simulink model "KitGewerk2_v1_4"  (R2014a)
settings: Solver=ode3  StartTime=0.0  StopTime=inf  FixedStep=0.005  RelTol=1e-3
undefined symbols (not defined in the file or in its folder): Com1, none
libraries: slrtlib x14, dspswit3 x1, xpcseriallib x1
(part 1 of 2)
CloseFcn:
  | rtwprivate ssgencode ModelCloseRequest Robotino_Strecke_reall_2009
settings Model: SimulationMode=external  BufferReuse=off  Creator=atlabor  LastModifiedBy=atlabor
settings SolverCC: EnableConcurrentExecution=on
settings DataIOCC: LimitDataPoints=off  SignalLoggingSaveFormat=ModelDataLogs
settings OptimizationCC: BlockReduction=off  OptimizeBlockIOStorage=off  BufferReuse=off  GlobalBufferReuse=off  ExpressionFolding=off  ExpressionDepthLimit=2147483647  LocalBlockOutputs=off  InitFltsAndDblsToZero=on
settings DebuggingCC: SaveWithParameterizedLinksMsg=none  UnderspecifiedInitializationDetection=Classic  FcnCallInpInsideContextMsg=UseLocalSettings  StateNameClashWarn=warning
settings HardwareCC: ProdIntDivRoundTo=Zero  ProdEndianess=LittleEndian  ProdHWDeviceType=Generic->32-bit x86 compatible
settings SFSimCC: SimParseCustomCode=off
settings RTWCC: SystemTargetFile=slrt.tlc  TemplateMakefile=slrt_default_tmf  Description=Simulink Real-Time  ProcessScript=slrt_make_rtw_hook  RTWCompilerOptimization=On
settings SimulinkRealTimeCC: GeneratePreprocessorConditionals=Disable all  EnableShiftOperators=on

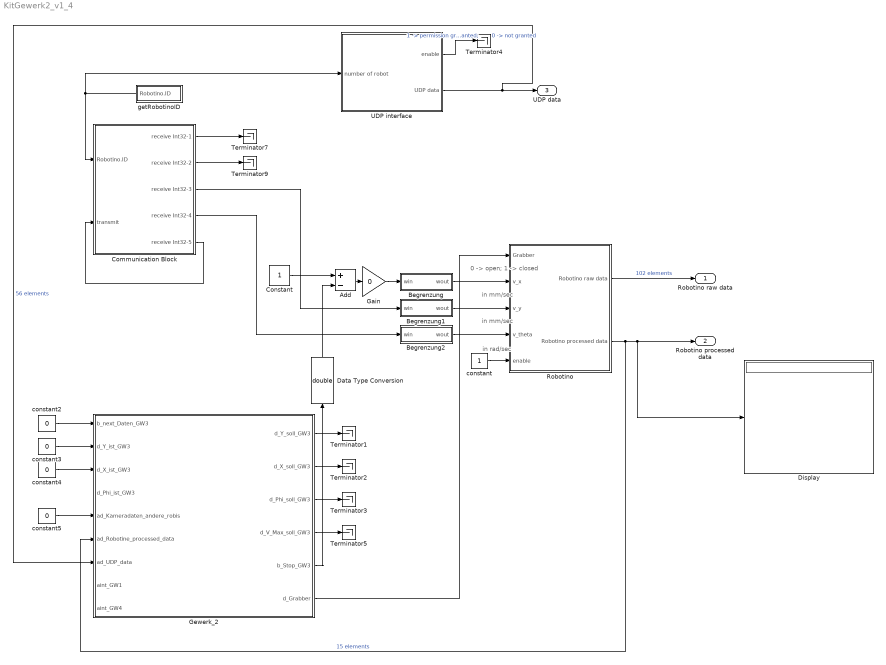
== system KitGewerk2_v1_4 ==
  note: 0 -> open; 1 -> closed
  note: in rad/sec
  note: in mm/sec
  note: in mm/sec
  Add : Sum  Inputs=+-
  Begrenzung : MATLAB Function  TreatAsAtomicUnit=on
  Begrenzung1 : MATLAB Function  TreatAsAtomicUnit=on
  Begrenzung2 : MATLAB Function  TreatAsAtomicUnit=on
  Communication Block : Subsystem
  Constant : Constant
  Data Type Conversion : DataTypeConversion  OutDataTypeStr=double
  Display : Display
  Gain : Gain  Gain=0
  Gewerk_2 : Subsystem
  Robotino : Subsystem
  Terminator{1..5,7,9} (7 alike) : Terminator
  UDP interface : Subsystem
  constant : Constant
  constant2 : Constant  Value=0  OutDataTypeStr=boolean
  constant3 : Constant  Value=0  OutDataTypeStr=double
  constant4 : Constant  Value=0
  constant5 : Constant  Value=0
  getRobotinoID : Subsystem
  Robotino raw data : Outport
  Robotino processed data : Outport  Port=2
  UDP data : Outport  Port=3
  wires:
  Robotino/1(Robotino raw data) -> Robotino raw data/1  "102 elements"
  Begrenzung1/1(wout) -> Robotino/3(v_y)
  Begrenzung/1(wout) -> Robotino/2(v_x)
  Communication Block/2(receive Int32-2) -> Terminator9/1
  UDP interface/1(enable) -> Terminator4/1  "1 -> permission granted;        0 -> not granted"
  constant/1 -> Robotino/5(enable)
  getRobotinoID/1(Robotino.ID) -> UDP interface/1(number of robot), Communication Block/1(Robotino.ID)
  Communication Block/5(receive Int32-5) -> Communication Block/2(transmit)
  Begrenzung2/1(wout) -> Robotino/4(v_theta)
  UDP interface/2(UDP data) -> Gewerk_2/7(ad_UDP_data), UDP data/1  "56 elements"
  Robotino/2(Robotino processed data) -> Gewerk_2/6(ad_Robotine_processed_data), Display/1, Robotino processed data/1  "15 elements"
  constant3/1 -> Gewerk_2/2(d_Y_ist_GW3)
  constant4/1 -> Gewerk_2/3(d_X_ist_GW3)
  constant5/1 -> Gewerk_2/5(ad_Kameradaten_andere_robis)
  Communication Block/3(receive Int32-3) -> Begrenzung1/1(win)
  Communication Block/4(receive Int32-4) -> Begrenzung2/1(win)
  Gewerk_2/1(d_Y_soll_GW3) -> Terminator1/1
  Gewerk_2/2(d_X_soll_GW3) -> Terminator2/1
  Gewerk_2/3(d_Phi_soll_GW3) -> Terminator3/1
  Gewerk_2/4(d_V_Max_soll_GW3) -> Terminator5/1
  Communication Block/1(receive Int32-1) -> Terminator7/1
  Add/1 -> Gain/1
  Constant/1 -> Add/1
  constant2/1 -> Gewerk_2/1(b_next_Daten_GW3)
  Gain/1 -> Begrenzung/1(win)
  Gewerk_2/5(b_Stop_GW3) -> Data Type Conversion/1
  Gewerk_2/6(d_Grabber) -> Robotino/1(Grabber)
  Data Type Conversion/1 -> Add/2

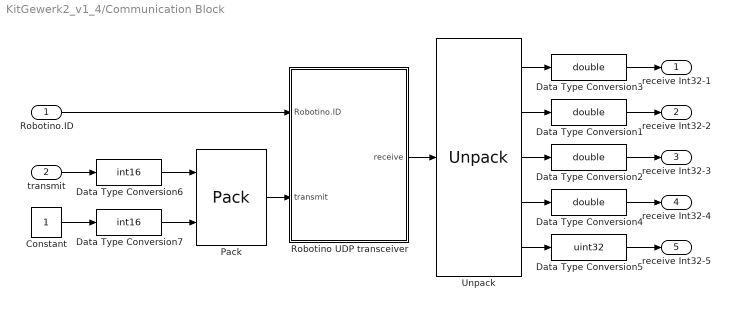
== system KitGewerk2_v1_4/Communication Block ==
  Robotino.ID : Inport
  transmit : Inport  Port=2
  Constant : Constant
  Data Type Conversion{1..4} (4 alike) : DataTypeConversion  OutDataTypeStr=double
  Data Type Conversion5 : DataTypeConversion  OutDataTypeStr=uint32
  Data Type Conversion6 : DataTypeConversion  OutDataTypeStr=int16
  Data Type Conversion7 : DataTypeConversion  OutDataTypeStr=int16
  Pack : slrtlib/UDP/Pack   datatypes={'int16','int16'}  byteAlign=1
  Robotino UDP transceiver : Subsystem
  Unpack : slrtlib/UDP/Unpack   dimensions={1, 1, 1, 1, 1}  datatypes={'int32','int32','int32','int32','int32'}  byteAlign=1
  receive Int32-1 : Outport
  receive Int32-2 : Outport  Port=2
  receive Int32-3 : Outport  Port=3
  receive Int32-4 : Outport  Port=4
  receive Int32-5 : Outport  Port=5
  wires:
  Unpack/1 -> Data Type Conversion3/1
  Unpack/5 -> Data Type Conversion5/1
  Unpack/2 -> Data Type Conversion1/1
  Unpack/3 -> Data Type Conversion2/1
  Unpack/4 -> Data Type Conversion4/1
  Data Type Conversion1/1 -> receive Int32-2/1
  Data Type Conversion2/1 -> receive Int32-3/1
  Data Type Conversion3/1 -> receive Int32-1/1
  Data Type Conversion4/1 -> receive Int32-4/1
  Data Type Conversion5/1 -> receive Int32-5/1
  transmit/1 -> Data Type Conversion6/1
  Pack/1 -> Robotino UDP transceiver/2(transmit)
  Data Type Conversion6/1 -> Pack/1
  Data Type Conversion7/1 -> Pack/2
  Constant/1 -> Data Type Conversion7/1
  Robotino.ID/1 -> Robotino UDP transceiver/1(Robotino.ID)
  Robotino UDP transceiver/1(receive) -> Unpack/1

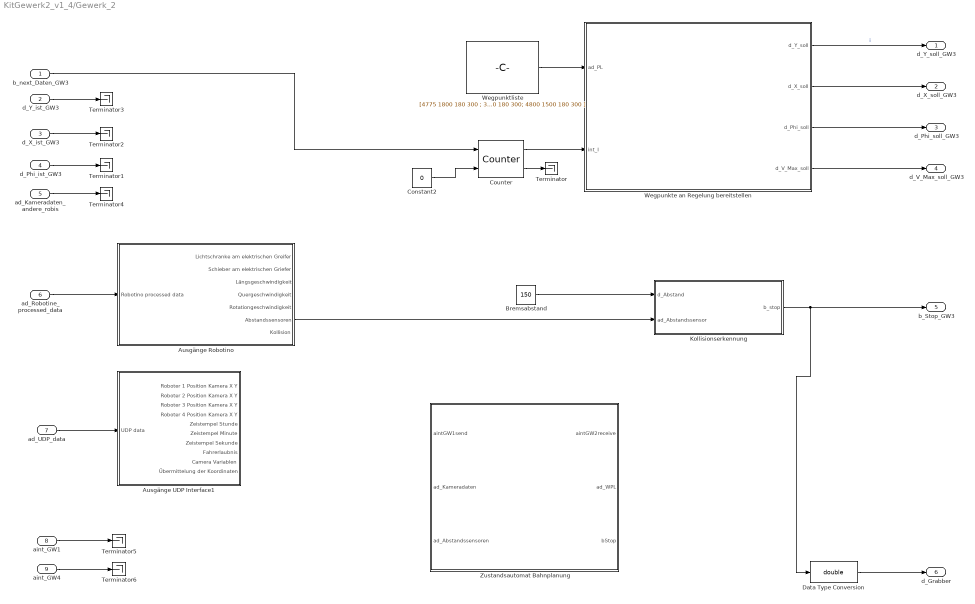
== system KitGewerk2_v1_4/Gewerk_2 ==
  b_next_Daten_GW3 : Inport  OutDataTypeStr=boolean
  d_Y_ist_GW3 : Inport  Port=2  OutDataTypeStr=double
  d_X_ist_GW3 : Inport  Port=3  OutDataTypeStr=double
  d_Phi_ist_GW3 : Inport  Port=4  OutDataTypeStr=double
  ad_Kameradaten_andere_robis : Inport  Port=5  OutDataTypeStr=double
  ad_Robotine_processed_data : Inport  Port=6
  ad_UDP_data : Inport  Port=7  OutDataTypeStr=double
  aint_GW1 : Inport  Port=8  OutDataTypeStr=boolean
  aint_GW4 : Inport  Port=9  OutDataTypeStr=boolean
  Ausgänge Robotino : Subsystem
  Ausgänge UDP Interface1 : Subsystem
  Bremsabstand : Constant  Value=150  OutDataTypeStr=double
  Constant2 : Constant  Value=0
  Counter : dspswit3/Counter  Direction=Up  CountEvent=Rising edge  CounterSize=User defined  MaxCount=16  InitialCount=0  Output=Count and Hit  HitValue=16  ResetInput=on  SamplesPerFrame=1  Ts=1  CntDtype=int32  HitDtype=Logical
  Data Type Conversion : DataTypeConversion  OutDataTypeStr=double
  Kollisionserkennung : MATLAB Function  TreatAsAtomicUnit=on
  Terminator{,1..6} (7 alike) : Terminator
  Wegpunkte an Regelung bereitstellen : MATLAB Function  TreatAsAtomicUnit=on
  Wegpunktliste : Constant  Value=[4775 1800 180 300 ; 3745 1800 180 300; 2540 2100 180 300; 2160 2100 180 300; 1678 1894 180 300; 1373 1846 180 300; 1155 1627 180 300; 1106 1321 180 300; 1246 1046 180 300; 1522 906 180 300; 1827 954 180 300; 2300 954 180 300; 2800 1500 180 300; 3300 1000 180 300; 3800 1500 180 300; 4300 1000 180 300; 4800 1500 180 300 ]  OutDataTypeStr=double
  Zustandsautomat Bahnplanung : Stateflow chart  TreatAsAtomicUnit=on
  d_Y_soll_GW3 : Outport  OutDataTypeStr=double
  d_X_soll_GW3 : Outport  Port=2  OutDataTypeStr=double
  d_Phi_soll_GW3 : Outport  Port=3  OutDataTypeStr=double
  d_V_Max_soll_GW3 : Outport  Port=4  OutDataTypeStr=double
  b_Stop_GW3 : Outport  Port=5  OutDataTypeStr=boolean
  d_Grabber : Outport  Port=6  OutDataTypeStr=double
  wires:
  d_Y_ist_GW3/1 -> Terminator3/1
  ad_Kameradaten_andere_robis/1 -> Terminator4/1
  d_Phi_ist_GW3/1 -> Terminator1/1
  d_X_ist_GW3/1 -> Terminator2/1
  Wegpunktliste/1 -> Wegpunkte an Regelung bereitstellen/1(ad_PL)
  Counter/1 -> Wegpunkte an Regelung bereitstellen/2(int_I)
  Wegpunkte an Regelung bereitstellen/2(d_X_soll) -> d_X_soll_GW3/1
  b_next_Daten_GW3/1 -> Counter/1
  Wegpunkte an Regelung bereitstellen/1(d_Y_soll) -> d_Y_soll_GW3/1  "i"
  Wegpunkte an Regelung bereitstellen/4(d_V_Max_soll) -> d_V_Max_soll_GW3/1
  Wegpunkte an Regelung bereitstellen/3(d_Phi_soll) -> d_Phi_soll_GW3/1
  Constant2/1 -> Counter/2
  Counter/2 -> Terminator/1
  Kollisionserkennung/1(b_stop) -> Data Type Conversion/1, b_Stop_GW3/1
  Ausgänge Robotino/6(Abstandssensoren) -> Kollisionserkennung/2(ad_Abstandssensor)
  Bremsabstand/1 -> Kollisionserkennung/1(d_Abstand)
  ad_Robotine_processed_data/1 -> Ausgänge Robotino/1(Robotino processed data)
  ad_UDP_data/1 -> Ausgänge UDP Interface1/1(UDP data)
  Data Type Conversion/1 -> d_Grabber/1
  aint_GW4/1 -> Terminator6/1
  aint_GW1/1 -> Terminator5/1

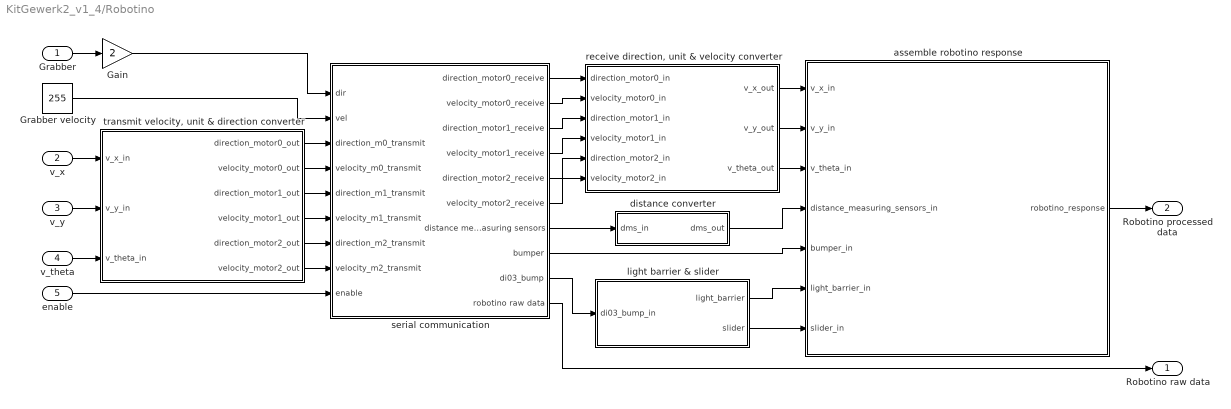
== system KitGewerk2_v1_4/Robotino ==
  Grabber : Inport
  v_x : Inport  Port=2
  v_y : Inport  Port=3
  v_theta : Inport  Port=4
  enable : Inport  Port=5
  Gain : Gain  Gain=2
  Grabber velocity : Constant  Value=255
  assemble robotino response : MATLAB Function  TreatAsAtomicUnit=on
  distance converter : MATLAB Function  TreatAsAtomicUnit=on
  light barrier & slider : MATLAB Function  TreatAsAtomicUnit=on
  "receive direction, unit & velocity converter" : MATLAB Function  TreatAsAtomicUnit=on
  serial communication : Subsystem
  "transmit velocity, unit & direction converter" : MATLAB Function  TreatAsAtomicUnit=on
  Robotino raw data : Outport
  Robotino processed data : Outport  Port=2
  wires:
  "transmit velocity, unit & direction converter"/1(direction_motor0_out) -> serial communication/3(direction_m0_transmit)
  "transmit velocity, unit & direction converter"/2(velocity_motor0_out) -> serial communication/4(velocity_m0_transmit)
  "transmit velocity, unit & direction converter"/3(direction_motor1_out) -> serial communication/5(direction_m1_transmit)
  "transmit velocity, unit & direction converter"/4(velocity_motor1_out) -> serial communication/6(velocity_m1_transmit)
  "transmit velocity, unit & direction converter"/5(direction_motor2_out) -> serial communication/7(direction_m2_transmit)
  "transmit velocity, unit & direction converter"/6(velocity_motor2_out) -> serial communication/8(velocity_m2_transmit)
  v_x/1 -> "transmit velocity, unit & direction converter"/1(v_x_in)
  v_y/1 -> "transmit velocity, unit & direction converter"/2(v_y_in)
  v_theta/1 -> "transmit velocity, unit & direction converter"/3(v_theta_in)
  "receive direction, unit & velocity converter"/2(v_y_out) -> assemble robotino response/2(v_y_in)
  enable/1 -> serial communication/9(enable)
  serial communication/1(direction_motor0_receive) -> "receive direction, unit & velocity converter"/1(direction_motor0_in)
  serial communication/7(distance measuring sensors) -> distance converter/1(dms_in)
  serial communication/10(robotino raw data) -> Robotino raw data/1
  serial communication/9(di03_bump) -> light barrier & slider/1(di03_bump_in)
  "receive direction, unit & velocity converter"/1(v_x_out) -> assemble robotino response/1(v_x_in)
  "receive direction, unit & velocity converter"/3(v_theta_out) -> assemble robotino response/3(v_theta_in)
  assemble robotino response/1(robotino_response) -> Robotino processed data/1
  Grabber/1 -> Gain/1
  Gain/1 -> serial communication/1(dir)
  distance converter/1(dms_out) -> assemble robotino response/4(distance_measuring_sensors_in)
  light barrier & slider/2(slider) -> assemble robotino response/7(slider_in)
  light barrier & slider/1(light_barrier) -> assemble robotino response/6(light_barrier_in)
  serial communication/8(bumper) -> assemble robotino response/5(bumper_in)
  serial communication/2(velocity_motor0_receive) -> "receive direction, unit & velocity converter"/2(velocity_motor0_in)
  serial communication/3(direction_motor1_receive) -> "receive direction, unit & velocity converter"/3(direction_motor1_in)
  serial communication/4(velocity_motor1_receive) -> "receive direction, unit & velocity converter"/4(velocity_motor1_in)
  serial communication/5(direction_motor2_receive) -> "receive direction, unit & velocity converter"/5(direction_motor2_in)
  serial communication/6(velocity_motor2_receive) -> "receive direction, unit & velocity converter"/6(velocity_motor2_in)
  Grabber velocity/1 -> serial communication/2(vel)

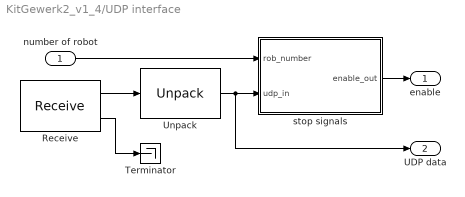
== system KitGewerk2_v1_4/UDP interface ==
  number of robot : Inport
  Receive : slrtlib/UDP/Receive   ipAddress=0.0.0.0  ipPort=25000  width=448  vblLen=off  sampletime=-1
  Terminator : Terminator
  Unpack : slrtlib/UDP/Unpack   dimensions={[56]}  datatypes={'double'}  byteAlign=1
  stop signals : MATLAB Function  TreatAsAtomicUnit=on
  enable : Outport
  UDP data : Outport  Port=2
  wires:
  Unpack/1 -> stop signals/2(udp_in), UDP data/1
  Receive/1 -> Unpack/1
  Receive/2 -> Terminator/1
  stop signals/1(enable_out) -> enable/1
  number of robot/1 -> stop signals/1(rob_number)

== system KitGewerk2_v1_4/getRobotinoID ==
  note: Executing only once at start after 10ms
  Step : Step  Time=0.01  SampleTime=0
  getIDfromFlash : Subsystem
  Robotino.ID : Outport
  wires:
  Step/1 -> getIDfromFlash/Trigger
  getIDfromFlash/1(RobotinoID) -> Robotino.ID/1

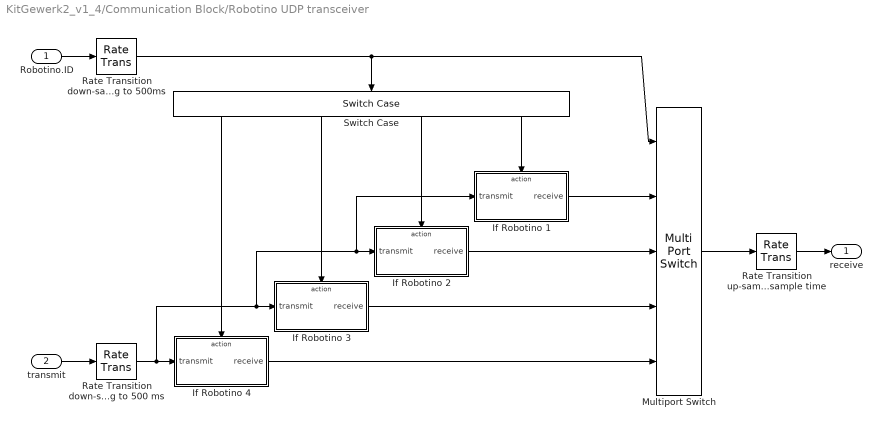
== system KitGewerk2_v1_4/Communication Block/Robotino UDP transceiver ==
  Robotino.ID : Inport
  transmit : Inport  Port=2
  If Robotino 1 : Subsystem  TreatAsAtomicUnit=on
  If Robotino 2 : Subsystem  TreatAsAtomicUnit=on
  If Robotino 3 : Subsystem  TreatAsAtomicUnit=on
  If Robotino 4 : Subsystem  TreatAsAtomicUnit=on
  Multiport Switch : MultiPortSwitch  Inputs=4
  Rate Transition down-sampling to 500 ms : RateTransition  OutPortSampleTime=0.5
  Rate Transition down-sampling to 500ms : RateTransition  OutPortSampleTime=0.5
  Rate Transition up-sampling to fundamental sample time : RateTransition
  Switch Case : SwitchCase  CaseConditions={4,3,2,1}  ShowDefaultCase=off
  receive : Outport
  wires:
  Switch Case/1 -> If Robotino 4/Action
  Switch Case/2 -> If Robotino 3/Action
  Switch Case/3 -> If Robotino 2/Action
  Switch Case/4 -> If Robotino 1/Action
  Multiport Switch/1 -> Rate Transition up-sampling to fundamental sample time/1
  If Robotino 1/1(receive) -> Multiport Switch/2
  If Robotino 3/1(receive) -> Multiport Switch/4
  If Robotino 2/1(receive) -> Multiport Switch/3
  If Robotino 4/1(receive) -> Multiport Switch/5
  transmit/1 -> Rate Transition down-sampling to 500 ms/1
  Rate Transition up-sampling to fundamental sample time/1 -> receive/1
  Rate Transition down-sampling to 500 ms/1 -> If Robotino 4/1(transmit), If Robotino 3/1(transmit), If Robotino 2/1(transmit), If Robotino 1/1(transmit)
  Robotino.ID/1 -> Rate Transition down-sampling to 500ms/1
  Rate Transition down-sampling to 500ms/1 -> Switch Case/1, Multiport Switch/1

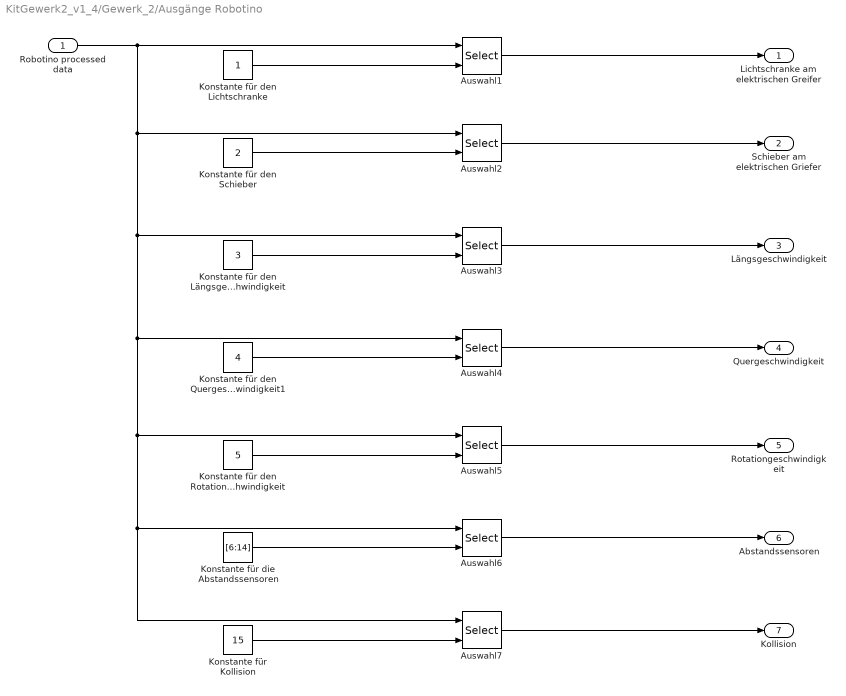
== system KitGewerk2_v1_4/Gewerk_2/Ausgänge Robotino ==
  Robotino processed data : Inport
  Auswahl{1..7} (7 alike) : Selector  InputPortWidth=15  IndexOptions=Index vector (port)  Indices=[1 3]
  "Konstante für Kollision " : Constant  Value=15
  Konstante für den Lichtschranke : Constant
  Konstante für den Längsgeschwindigkeit : Constant  Value=3
  Konstante für den Quergeschwindigkeit1 : Constant  Value=4
  Konstante für den Rotationegeschwindigkeit : Constant  Value=5
  Konstante für den Schieber : Constant  Value=2
  Konstante für die Abstandssensoren : Constant  Value=[6:14]
  Lichtschranke am elektrischen Greifer : Outport
  "Schieber am elektrischen Griefer " : Outport  Port=2
  "Längsgeschwindigkeit " : Outport  Port=3
  Quergeschwindigkeit : Outport  Port=4
  "Rotationgeschwindigkeit " : Outport  Port=5
  Abstandssensoren : Outport  Port=6
  Kollision : Outport  Port=7
  wires:
  Auswahl1/1 -> Lichtschranke am elektrischen Greifer/1
  Robotino processed data/1 -> Auswahl1/1, Auswahl5/1, Auswahl7/1, Auswahl6/1, Auswahl4/1, Auswahl3/1, Auswahl2/1
  Konstante für den Lichtschranke/1 -> Auswahl1/2
  Konstante für den Schieber/1 -> Auswahl2/2
  Auswahl2/1 -> "Schieber am elektrischen Griefer "/1
  Konstante für den Längsgeschwindigkeit/1 -> Auswahl3/2
  Auswahl3/1 -> "Längsgeschwindigkeit "/1
  Konstante für den Quergeschwindigkeit1/1 -> Auswahl4/2
  Auswahl4/1 -> Quergeschwindigkeit/1
  Auswahl5/1 -> "Rotationgeschwindigkeit "/1
  Konstante für den Rotationegeschwindigkeit/1 -> Auswahl5/2
  Konstante für die Abstandssensoren/1 -> Auswahl6/2
  Auswahl6/1 -> Abstandssensoren/1
  Auswahl7/1 -> Kollision/1
  "Konstante für Kollision "/1 -> Auswahl7/2

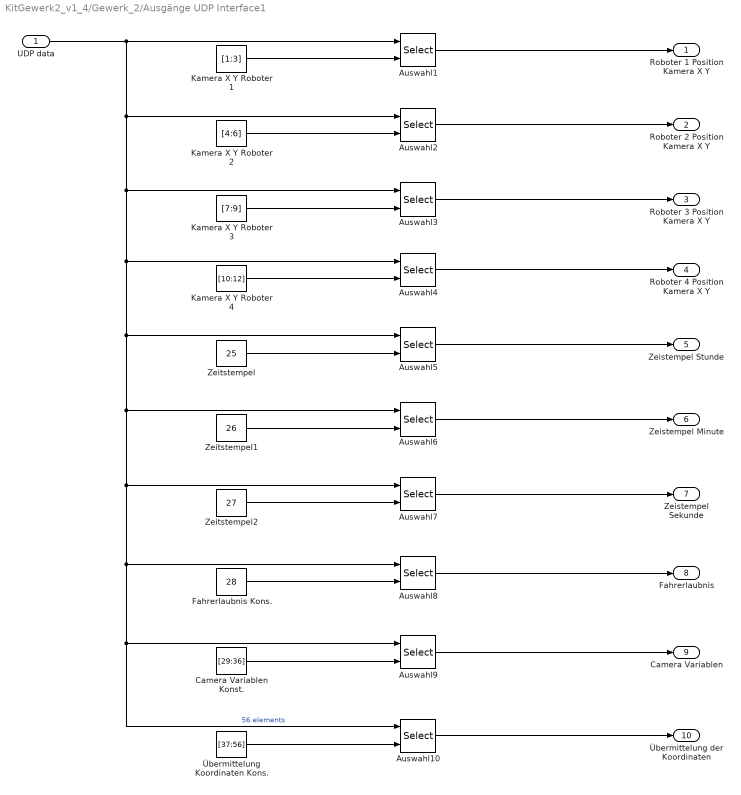
== system KitGewerk2_v1_4/Gewerk_2/Ausgänge UDP Interface1 ==
  UDP data : Inport
  Auswahl{1..10} (10 alike) : Selector  InputPortWidth=56  IndexOptions=Index vector (port)  Indices=[1 3]
  Camera Variablen Konst. : Constant  Value=[29:36]
  Fahrerlaubnis Kons. : Constant  Value=28
  Kamera X Y Roboter 1 : Constant  Value=[1:3]
  Kamera X Y Roboter 2 : Constant  Value=[4:6]
  Kamera X Y Roboter 3 : Constant  Value=[7:9]
  Kamera X Y Roboter 4 : Constant  Value=[10:12]
  Zeitstempel : Constant  Value=25
  Zeitstempel1 : Constant  Value=26
  Zeitstempel2 : Constant  Value=27
  Übermittelung Koordinaten Kons. : Constant  Value=[37:56]
  Roboter 1 Position Kamera X Y : Outport
  Roboter 2 Position Kamera X Y : Outport  Port=2
  Roboter 3 Position Kamera X Y : Outport  Port=3
  Roboter 4 Position Kamera X Y : Outport  Port=4
  Zeistempel Stunde : Outport  Port=5
  Zeistempel Minute : Outport  Port=6
  Zeistempel Sekunde : Outport  Port=7
  Fahrerlaubnis : Outport  Port=8
  Camera Variablen : Outport  Port=9
  Übermittelung der Koordinaten : Outport  Port=10
  wires:
  Kamera X Y Roboter 1/1 -> Auswahl1/2
  Kamera X Y Roboter 2/1 -> Auswahl2/2
  Kamera X Y Roboter 3/1 -> Auswahl3/2
  Kamera X Y Roboter 4/1 -> Auswahl4/2
  Auswahl1/1 -> Roboter 1 Position Kamera X Y/1
  Auswahl3/1 -> Roboter 3 Position Kamera X Y/1
  Auswahl2/1 -> Roboter 2 Position Kamera X Y/1
  Auswahl4/1 -> Roboter 4 Position Kamera X Y/1
  Zeitstempel/1 -> Auswahl5/2
  Auswahl5/1 -> Zeistempel Stunde/1
  Zeitstempel1/1 -> Auswahl6/2
  Auswahl6/1 -> Zeistempel Minute/1
  Zeitstempel2/1 -> Auswahl7/2
  Auswahl7/1 -> Zeistempel Sekunde/1
  Fahrerlaubnis Kons./1 -> Auswahl8/2
  Auswahl8/1 -> Fahrerlaubnis/1
  Camera Variablen Konst./1 -> Auswahl9/2
  Auswahl9/1 -> Camera Variablen/1
  UDP data/1 -> Auswahl2/1, Auswahl10/1, Auswahl9/1, Auswahl8/1, Auswahl7/1, Auswahl6/1, Auswahl5/1, Auswahl4/1, Auswahl3/1, Auswahl1/1  "56 elements"
  Übermittelung Koordinaten Kons./1 -> Auswahl10/2
  Auswahl10/1 -> Übermittelung der Koordinaten/1

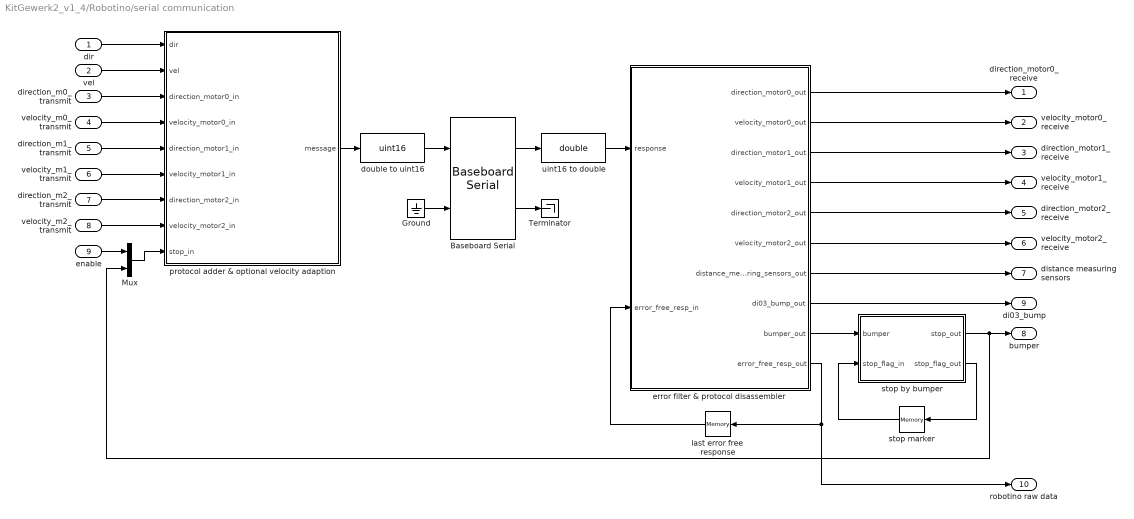
== system KitGewerk2_v1_4/Robotino/serial communication ==
  dir : Inport
  vel : Inport  Port=2
  direction_m0_transmit : Inport  Port=3
  velocity_m0_transmit : Inport  Port=4
  direction_m1_transmit : Inport  Port=5
  velocity_m1_transmit : Inport  Port=6
  direction_m2_transmit : Inport  Port=7
  velocity_m2_transmit : Inport  Port=8
  enable : Inport  Port=9
  Baseboard Serial : xpcseriallib/Mainboard/Baseboard Serial  group=Transmit Setup  port=2  irqnum=4  saddr1=0x3f8  saddr2=0x3e8  config=Com1/none  baud1=115200  parity1=None  ndata1=8  nstop1=1  fifomode1=16 deep  rlevel1=almost full  automode1=off  xmtfifosize1=10240  xmtdatatype1=count+16 bit uint  rcvfifosize1=10240  rcvmaxread1=101  rcvminread1=1  rcvusedelim1=on  rcvdelim1=99  rcvdatatype1=count+16 bit uint  rcvsampletime1=-1  baud2=115200  parity2=None  ndata2=8  nstop2=1  fifomode2=16 deep  rlevel2=almost full  automode2=off  xmtfifosize2=10240  xmtdatatype2=count+16 bit uint  rcvfifosize2=10240  rcvmaxread2=101  rcvminread2=1  rcvusedelim2=on  rcvdelim2=99  rcvdatatype2=count+16 bit uint  rcvsampletime2=-1
      link override FIFO read 1: maxsize=101  minsize=1  usedelimiter=on  delimiter=99  outputtype=count+16 bit uint  sampletime=dt / 2
      link override FIFO read 2: maxsize=101  minsize=1  usedelimiter=on  delimiter=99  outputtype=count+16 bit uint  sampletime=dt / 2
      link override FIFO write 1: size=1024  inputtype=count+16 bit uint  sampletime=-1  id=XMT channel 1, IRQ 4
      link override FIFO write 2: size=1024  inputtype=8 bit uint null terminated  id=XMT channel 2, IRQ 4
      link override Setup1: baud=115200  width=8  nstop=1  parity=None  fmode=16 deep  rlevel=half full  ctsmode=off
      link override Setup2: baud=4800  width=8  nstop=1  parity=None  fmode=16 deep  rlevel=half full  ctsmode=off
  Ground : Ground
  Mux : Mux  Inputs=2
  Terminator : Terminator
  double to uint16 : DataTypeConversion  OutDataTypeStr=uint16  RndMeth=Nearest
  error filter & protocol disassembler : MATLAB Function  TreatAsAtomicUnit=on
  last error free response : Memory  X0=[zeros(1,102)]
  protocol adder & optional velocity adaption : MATLAB Function  TreatAsAtomicUnit=on
  stop by bumper : MATLAB Function  TreatAsAtomicUnit=on
  stop marker : Memory  X0=[zeros(1,3)]
  uint16 to double : DataTypeConversion  OutDataTypeStr=double  RndMeth=Nearest
  direction_motor0_receive : Outport
  velocity_motor0_receive : Outport  Port=2
  direction_motor1_receive : Outport  Port=3
  velocity_motor1_receive : Outport  Port=4
  direction_motor2_receive : Outport  Port=5
  velocity_motor2_receive : Outport  Port=6
  distance measuring sensors : Outport  Port=7
  bumper : Outport  Port=8
  di03_bump : Outport  Port=9
  robotino raw data : Outport  Port=10
  wires:
  Ground/1 -> Baseboard Serial/2
  Baseboard Serial/2 -> Terminator/1
  double to uint16/1 -> Baseboard Serial/1
  protocol adder & optional velocity adaption/1(message) -> double to uint16/1
  stop marker/1 -> stop by bumper/2(stop_flag_in)
  stop by bumper/2(stop_flag_out) -> stop marker/1
  last error free response/1 -> error filter & protocol disassembler/2(error_free_resp_in)
  error filter & protocol disassembler/10(error_free_resp_out) -> last error free response/1, robotino raw data/1
  error filter & protocol disassembler/1(direction_motor0_out) -> direction_motor0_receive/1
  error filter & protocol disassembler/2(velocity_motor0_out) -> velocity_motor0_receive/1
  error filter & protocol disassembler/3(direction_motor1_out) -> direction_motor1_receive/1
  error filter & protocol disassembler/4(velocity_motor1_out) -> velocity_motor1_receive/1
  direction_m0_transmit/1 -> protocol adder & optional velocity adaption/3(direction_motor0_in)
  error filter & protocol disassembler/5(direction_motor2_out) -> direction_motor2_receive/1
  velocity_m0_transmit/1 -> protocol adder & optional velocity adaption/4(velocity_motor0_in)
  error filter & protocol disassembler/6(velocity_motor2_out) -> velocity_motor2_receive/1
  direction_m1_transmit/1 -> protocol adder & optional velocity adaption/5(direction_motor1_in)
  velocity_m1_transmit/1 -> protocol adder & optional velocity adaption/6(velocity_motor1_in)
  direction_m2_transmit/1 -> protocol adder & optional velocity adaption/7(direction_motor2_in)
  velocity_m2_transmit/1 -> protocol adder & optional velocity adaption/8(velocity_motor2_in)
  error filter & protocol disassembler/9(bumper_out) -> stop by bumper/1(bumper)
  stop by bumper/1(stop_out) -> bumper/1, Mux/2
  error filter & protocol disassembler/7(distance_measuring_sensors_out) -> distance measuring sensors/1
  Baseboard Serial/1 -> uint16 to double/1
  uint16 to double/1 -> error filter & protocol disassembler/1(response)
  enable/1 -> Mux/1
  dir/1 -> protocol adder & optional velocity adaption/1(dir)
  vel/1 -> protocol adder & optional velocity adaption/2(vel)
  Mux/1 -> protocol adder & optional velocity adaption/9(stop_in)
  error filter & protocol disassembler/8(di03_bump_out) -> di03_bump/1

== system KitGewerk2_v1_4/getRobotinoID/getIDfromFlash ==
  Trigger : TriggerPort
  From File : slrtlib/Target Management/From File   filename='robotino.id'  dataSize=8  bufSize=2000  readSize=512  EOFOption=Seek to beginning  sampTime=-1  show2ports=off
  Unpack : slrtlib/UDP/Unpack   dimensions={[1]}  datatypes={'double'}  byteAlign=1
  RobotinoID : Outport
  wires:
  From File/1 -> Unpack/1
  Unpack/1 -> RobotinoID/1

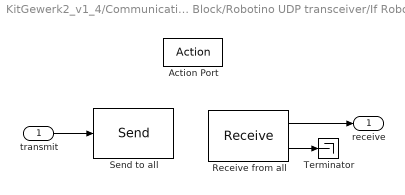
== system KitGewerk2_v1_4/Communication Block/Robotino UDP transceiver/If Robotino 1 ==
  transmit : Inport
  Action Port : ActionPort  ActionType=case
  Receive from all : slrtlib/UDP/Receive   ipAddress=0.0.0.0  ipPort=25011  width=20  vblLen=off  sampletime=-1
  Send to all : slrtlib/UDP/Send   ipAddress=255.255.255.255  ipPort=25010  localPort=-1  vblLen=off  sampletime=-1
  Terminator : Terminator
  receive : Outport
  wires:
  Receive from all/1 -> receive/1
  Receive from all/2 -> Terminator/1
  transmit/1 -> Send to all/1

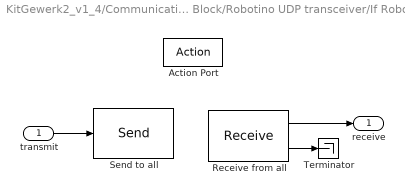
== system KitGewerk2_v1_4/Communication Block/Robotino UDP transceiver/If Robotino 2 ==
  transmit : Inport
  Action Port : ActionPort  ActionType=case
  Receive from all : slrtlib/UDP/Receive   ipAddress=0.0.0.0  ipPort=25012  width=20  vblLen=off  sampletime=-1
  Send to all : slrtlib/UDP/Send   ipAddress=255.255.255.255  ipPort=25020  localPort=-1  vblLen=off  sampletime=-1
  Terminator : Terminator
  receive : Outport
  wires:
  Receive from all/1 -> receive/1
  Receive from all/2 -> Terminator/1
  transmit/1 -> Send to all/1

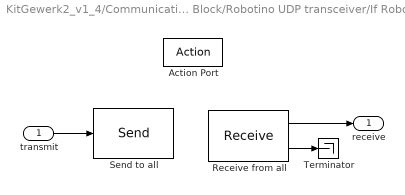
== system KitGewerk2_v1_4/Communication Block/Robotino UDP transceiver/If Robotino 3 ==
  transmit : Inport
  Action Port : ActionPort  ActionType=case
  Receive from all : slrtlib/UDP/Receive   ipAddress=0.0.0.0  ipPort=25013  width=20  vblLen=off  sampletime=-1
  Send to all : slrtlib/UDP/Send   ipAddress=255.255.255.255  ipPort=25030  localPort=-1  vblLen=off  sampletime=-1
  Terminator : Terminator
  receive : Outport
  wires:
  Receive from all/1 -> receive/1
  Receive from all/2 -> Terminator/1
  transmit/1 -> Send to all/1

== system KitGewerk2_v1_4/Communication Block/Robotino UDP transceiver/If Robotino 4 ==
  transmit : Inport
  Action Port : ActionPort  ActionType=case
  Receive from all : slrtlib/UDP/Receive   ipAddress=0.0.0.0  ipPort=25014  width=20  vblLen=off  sampletime=-1
  Send to all : slrtlib/UDP/Send   ipAddress=255.255.255.255  ipPort=25040  localPort=-1  vblLen=off  sampletime=-1
  Terminator : Terminator
  receive : Outport
  wires:
  Receive from all/1 -> receive/1
  Receive from all/2 -> Terminator/1
  transmit/1 -> Send to all/1

== matlab function KitGewerk2_v1_4/Robotino/transmit velocity, unit & direction converter ==
  settings: sampleTime=2*dtpc
  data: direction_motor0_out output; velocity_motor0_out output; direction_motor1_out output; velocity_motor1_out output; direction_motor2_out output; velocity_motor2_out output; v_x_in input; v_y_in input; v_theta_in input
%%%%%%%%%%%%%%%%%%%%%%%%%%%%%%%%%%%%%%%%%%%%%%%%%%%%%%%%%%%%%%%%%%%%%%%%%%%
% conversion from positive and/or negative longitudinal, lateral and      %
% rotational velocities (in milimeters per second) to three separate      %
% positive motor velocities (resolution: 1Byte) and their rotation        %
% direction                                                               %
%                                                                         %
% inputs:  v_x_in (longitudinal velocity in milimeters per second),       %
%          v_y_in (lateral velocity in milimeters per second),            %
%          v_theta_in (rotational velocity in milimeters per second)      %
% outputs: direction_motor0_out (rotating direction of motor0             %
%          (0 := counter-clockwise; 2 := clockwise)),                     %
%          velocity_motor0_out (from 0 to 255),                           %
%          direction_motor1_out (rotating direction of motor1             %
%          (0 := counter-clockwise; 2 := clockwise)),                     %
%          velocity_motor1_out (from 0 to 255),                           %
%          direction_motor2_out (rotating direction of motor2             %
%          (0 := counter-clockwise; 2 := clockwise)),                     %
%          velocity_motor2_out (from 0 to 255)                            %
%%%%%%%%%%%%%%%%%%%%%%%%%%%%%%%%%%%%%%%%%%%%%%%%%%%%%%%%%%%%%%%%%%%%%%%%%%%
function [direction_motor0_out, velocity_motor0_out, ...
          direction_motor1_out, velocity_motor1_out, ...
          direction_motor2_out, velocity_motor2_out] ...
                                          = fcn(v_x_in, v_y_in, v_theta_in)
%%%%%%%%%%%%%%%%%%%%%%%%%%%%%%%%%%%%%%%%%%%%%%%%%%%%%%%%%%%%%%%%%%%%%%
% conversion from longitudinal, lateral & rotational velocity to the %
% three separate motor velocities                                    %
%%%%%%%%%%%%%%%%%%%%%%%%%%%%%%%%%%%%%%%%%%%%%%%%%%%%%%%%%%%%%%%%%%%%%%
v0 = (-v_x_in * cosd(30)) + ( v_y_in * cosd(60)) + (v_theta_in * 135);
v1 =                      + (-v_y_in)            + (v_theta_in * 135);
v2 = ( v_x_in * cosd(30)) + ( v_y_in * cosd(60)) + (v_theta_in * 135);

%%%%%%%%%%%%%%%%%%%%%%%%%%%%%%%%%%%%%%%%%%%%%%%%%%%%%%%%%%%%%%%%%%%%%
% conversion of the separate motor velocities from millimeters to a %
% value between -255 and 255                                        %
%%%%%%%%%%%%%%%%%%%%%%%%%%%%%%%%%%%%%%%%%%%%%%%%%%%%%%%%%%%%%%%%%%%%%
f = 1 / 7.02;
v0 = v0 * f;
v1 = v1 * f;
v2 = v2 * f;

%%%%%%%%%%%%%%%%%%%%%%%%%%%%%%%%%%%%%%%%%%%%%%%%%%%%%%%%%%%%%%%%%%%%
% division of motor velocities into absolute velocity and rotating %
% direction                                                        %
%%%%%%%%%%%%%%%%%%%%%%%%%%%%%%%%%%%%%%%%%%%%%%%%%%%%%%%%%%%%%%%%%%%%
if v0 < 0
    direction_motor0_out =  0;
    velocity_motor0_out  = -v0;
else
    direction_motor0_out = 2;
    velocity_motor0_out  = v0;
end

if v1 < 0
    direction_motor1_out =  0;
    velocity_motor1_out  = -v1;
else
    direction_motor1_out = 2;
    velocity_motor1_out  = v1;
end

if v2 < 0
    direction_motor2_out =  0;
    velocity_motor2_out  = -v2;
else
    direction_motor2_out = 2;
    velocity_motor2_out  = v2;
end

== matlab function KitGewerk2_v1_4/Robotino/serial communication/protocol adder & optional velocity adaption ==
  settings: sampleTime=2*dtpc
  data: dir input; vel input; direction_motor0_in input; velocity_motor0_in input; direction_motor1_in input; velocity_motor1_in input; direction_motor2_in input; velocity_motor2_in input; stop_in input; message output
%%%%%%%%%%%%%%%%%%%%%%%%%%%%%%%%%%%%%%%%%%%%%%%%%%%%%%%%%%%%%%%%%%%%%%%%%%%
% parameterising the 'PC104 to I/O-Board message' for serial line         %
% communication with control commands for the robotino motors             %
%                                                                         %
% optional: velocity adaption as soon as at least one motor is near the   %
%           speed limit                                                   %
%                                                                         %
% inputs: rotating directions and velocities of the three motors          %
% output: vector containing the 'PC104 to I/O-Board message' for serial   %
%         line communication                                              %
%%%%%%%%%%%%%%%%%%%%%%%%%%%%%%%%%%%%%%%%%%%%%%%%%%%%%%%%%%%%%%%%%%%%%%%%%%%
function message = fcn(dir, vel, direction_motor0_in, velocity_motor0_in, ...
                       direction_motor1_in, velocity_motor1_in, ...
                       direction_motor2_in, velocity_motor2_in, stop_in)
%%%%%%%%%%%%%%%%%%%%%%%%%%%%%%
% optional velocity adaption %
%%%%%%%%%%%%%%%%%%%%%%%%%%%%%%
vmax = 175;                                               % v_motor_dez_max

if velocity_motor0_in > vmax
    velocity_motor0_tf = velocity_motor0_in;
    
    velocity_motor0_in = vmax;
    velocity_motor1_in = vmax * velocity_motor1_in / velocity_motor0_tf;
    velocity_motor2_in = vmax * velocity_motor2_in / velocity_motor0_tf;
end

if velocity_motor1_in > vmax
    velocity_motor1_tf = velocity_motor1_in;
    
    velocity_motor0_in = vmax * velocity_motor0_in / velocity_motor1_tf;
    velocity_motor1_in = vmax;
    velocity_motor2_in = vmax * velocity_motor2_in / velocity_motor1_tf;
end

if velocity_motor2_in > vmax
    velocity_motor2_tf = velocity_motor2_in;
    
    velocity_motor0_in = vmax * velocity_motor0_in / velocity_motor2_tf;
    velocity_motor1_in = vmax * velocity_motor1_in / velocity_motor2_tf;
    velocity_motor2_in = vmax;
end
%%%%%%%%%%%%%%%%%%%%%%%%%%%%%%%%%%%%%%%%%%%%%%%%%%%%%%%%%%%%%%%%%%%%%%
% vector containing the 'PC104 to I/O-Board message' for serial line %
% communication                                                      %
%%%%%%%%%%%%%%%%%%%%%%%%%%%%%%%%%%%%%%%%%%%%%%%%%%%%%%%%%%%%%%%%%%%%%%
message = [47, abs('REC'), 5, min(stop_in), direction_motor0_in, ...
           velocity_motor0_in, zeros(1, 4), 255, 255, 255, ...
           min(stop_in), direction_motor1_in, velocity_motor1_in, ...
           zeros(1, 4), 255, 255, 255, min(stop_in), ...
           direction_motor2_in, velocity_motor2_in, zeros(1, 4), 255, ...
           255, 255, 1, dir, vel, zeros(1, 4), 255, 255, 255, abs('rec')].';

== matlab function KitGewerk2_v1_4/UDP interface/stop signals ==
  data: rob_number input; udp_in input; enable_out output
%%%%%%%%%%%%%%%%%%%%%%%%%%%%%%%%%%%%%%%%%%%%%%%%%%%%%%%%%%%%%%%%%%%%%%%%%%%
% Leads the enable command through. The enable command turns the Robotino %
% inputs to selectable form.                                              %
%                                                                         %
% input: udp_in (vector of 56 elements containing the data sent by the    %
%                camera-model)                                            %
% outputs: enable_out (1 = inputs are in selectable form;                 %
%                      0 = inputs are set to 0)                           %
%          udp_out (vector of 56 elements containing the data sent by the %
%                   camera-model)                                         %
%%%%%%%%%%%%%%%%%%%%%%%%%%%%%%%%%%%%%%%%%%%%%%%%%%%%%%%%%%%%%%%%%%%%%%%%%%%
function enable_out  = fcn(rob_number, udp_in)
enable_out = [0, 0];
if (udp_in(rob_number * 3 - 2) <= 0) && ...
   (udp_in(rob_number * 3 - 1) <= 0) && (udp_in(rob_number * 3) <= 0)
    enable_out(1) = 0;
else
    enable_out(1) = 1;
end
enable_out(2) = udp_in(28);

== matlab function KitGewerk2_v1_4/Robotino/serial communication/error filter & protocol disassembler ==
  settings: sampleTime=dtpc/2
  data: response input; error_free_resp_in input; direction_motor0_out output; velocity_motor0_out output; direction_motor1_out output; velocity_motor1_out output; direction_motor2_out output; velocity_motor2_out output; distance_measuring_sensors_out output; di03_bump_out output; bumper_out output; error_free_resp_out output
%%%%%%%%%%%%%%%%%%%%%%%%%%%%%%%%%%%%%%%%%%%%%%%%%%%%%%%%%%%%%%%%%%%%%%%%%%%
% Error check of the 'I/O-Board to PC104 message' and filtering of this   %
% defective response: Substitute defective message by the last error free %
% message.                                                                %
% Saving of the rotating direction, velocity, shaft position and running  %
% time of the three motors. Combining all shaft positions in a vector.    %
% Combining all running times in a vector.                                %
% Saving of the three bumper bytes indicating a collision in a vector.    %
% Saving the values of the nine distance measuring IR-sensors in a vector.%
%                                                                         %
% inputs: response (actual 'I/O-Board to PC104 message')(vector 102       %
%                   elements)                                             %
%         error_free_resp_in (last error free 'I/O-Board to PC104         %
%                             message')                                   %
% outputs: directions and velocities of the three motors                  %
%          motor_positions_out (shaft positions of the three motors)      %
%                              (vector 12 elements)                       %
%          time_bytes_out (running times of the three motors)             %
%                         (vector 9 elements)                             %
%          distance_measuring_sensors_out (values of the nine IR-sensors) %
%                                         (vector 9 elements)             %
%          bumper_out (vector 3 elements)                                 %
%          error_free_resp_out (error free 'I/O-Board to PC104 message')  %
%                              (vector 102 elements)                      %
%%%%%%%%%%%%%%%%%%%%%%%%%%%%%%%%%%%%%%%%%%%%%%%%%%%%%%%%%%%%%%%%%%%%%%%%%%%
function [direction_motor0_out, velocity_motor0_out, ...
          direction_motor1_out, velocity_motor1_out, ...
          direction_motor2_out, velocity_motor2_out, ...
          distance_measuring_sensors_out, di03_bump_out, bumper_out, ...
          error_free_resp_out] = fcn(response, error_free_resp_in)
%           motor_positions_out, time_bytes_out, ...)
      
%%%%%%%%%%%%%%%%%%%%%%%%%%%%%%%%%%%%%%%%%%%%%%%%%%%%%
% filtering defective 'I/O-Board to PC104 messages' %
%%%%%%%%%%%%%%%%%%%%%%%%%%%%%%%%%%%%%%%%%%%%%%%%%%%%%
if (response(1) == 101) && (response(2) == 82) && (response(3) == 69) ...
   && (response(4) == 67) && (response(100) == 114) ...        % if the ...
   && (response(101) == 101) && (response(102) == 99)  % counter (101), ...
                        % the start (REC) and stop (rec) bytes are true ...
    error_free_resp_out = response;     % save the actual 'I/O-Board to ...
                                                           % PC104 message'
else                                                        % otherwise ...
    error_free_resp_out = error_free_resp_in;     % save the last error ...
                                        % free 'I/O-Board to PC104 message'
end

%%%%%%%%%%%%%%%%%%%%%%%%%%%%%%%%%%%%%%%%%%%%%%%%%%%%%%%%%%%%%%%%%%%%%%%%%%
% save rotating direction, velocity, shaft position and the running time %
% of motor0                                                              %
%%%%%%%%%%%%%%%%%%%%%%%%%%%%%%%%%%%%%%%%%%%%%%%%%%%%%%%%%%%%%%%%%%%%%%%%%%
direction_motor0_out  = error_free_resp_out(26);
velocity_motor0_out   = error_free_resp_out(27);
% position_motor0_byte1 = error_free_resp_out(28);
% position_motor0_byte2 = error_free_resp_out(29);
% position_motor0_byte3 = error_free_resp_out(30);
% position_motor0_byte4 = error_free_resp_out(31);
% time_motor0_byte1     = error_free_resp_out(34);
% time_motor0_byte2     = error_free_resp_out(35);
% time_motor0_byte3     = error_free_resp_out(36);

%%%%%%%%%%%%%%%%%%%%%%%%%%%%%%%%%%%%%%%%%%%%%%%%%%%%%%%%%%%%%%%%%%%%%%%%%%
% save rotating direction, velocity, shaft position and the running time %
% of motor1                                                              %
%%%%%%%%%%%%%%%%%%%%%%%%%%%%%%%%%%%%%%%%%%%%%%%%%%%%%%%%%%%%%%%%%%%%%%%%%%
direction_motor1_out  = error_free_resp_out(47);
velocity_motor1_out   = error_free_resp_out(48);
% position_motor1_byte1 = error_free_resp_out(49);
% position_motor1_byte2 = error_free_resp_out(50);
% position_motor1_byte3 = error_free_resp_out(51);
% position_motor1_byte4 = error_free_resp_out(52);
% time_motor1_byte1     = error_free_resp_out(55);
% time_motor1_byte2     = error_free_resp_out(56);
% time_motor1_byte3     = error_free_resp_out(57);

%%%%%%%%%%%%%%%%%%%%%%%%%%%%%%%%%%%%%%%%%%%%%%%%%%%%%%%%%%%%%%%%%%%%%%%%%%
% save rotating direction, velocity, shaft position and the running time %
% of motor2                                                              %
%%%%%%%%%%%%%%%%%%%%%%%%%%%%%%%%%%%%%%%%%%%%%%%%%%%%%%%%%%%%%%%%%%%%%%%%%%
direction_motor2_out  = error_free_resp_out(68);
velocity_motor2_out   = error_free_resp_out(69);
% position_motor2_byte1 = error_free_resp_out(70);
% position_motor2_byte2 = error_free_resp_out(71);
% position_motor2_byte3 = error_free_resp_out(72);
% position_motor2_byte4 = error_free_resp_out(73);
% time_motor2_byte1     = error_free_resp_out(76);
% time_motor2_byte2     = error_free_resp_out(77);
% time_motor2_byte3     = error_free_resp_out(78);

%%%%%%%%%%%%%%%%%%%%%%%%%%%%%%%%%%%%%%%%%%%
% save the three bumper bytes in a vector %
%%%%%%%%%%%%%%%%%%%%%%%%%%%%%%%%%%%%%%%%%%%
bumper_out = [error_free_resp_out(32), error_free_resp_out(53), ...
              error_free_resp_out(74)]';
          
%%%%%%%%%%%%%%%%%%%%%%%%%%%%%%%%%%%%%%%%%%%%%%%%%%%%%%%%%%%%%%%%%%%%%%
% save the values of the nine distance measuring sensors in a vector %
%%%%%%%%%%%%%%%%%%%%%%%%%%%%%%%%%%%%%%%%%%%%%%%%%%%%%%%%%%%%%%%%%%%%%%
distance_measuring_sensors_out = [error_free_resp_out(60), ...
                    error_free_resp_out(59), error_free_resp_out(44), ...
                    error_free_resp_out(39), error_free_resp_out(38), ...
                    error_free_resp_out(17), error_free_resp_out(18), ...
                    error_free_resp_out(23), error_free_resp_out(65)];
                
%%%%%%%%%%%%%%%%%%%%%%%%%%%%%%%%%%%%%%%%%%%%%%%%%%%%%%%%
% save positions of the three motor shafts in a vector %
%%%%%%%%%%%%%%%%%%%%%%%%%%%%%%%%%%%%%%%%%%%%%%%%%%%%%%%%
% motor_positions_out = [position_motor0_byte1, position_motor0_byte2, ...
%                        position_motor0_byte3, position_motor0_byte4, ...
%                        position_motor1_byte1, position_motor1_byte2, ...
%                        position_motor1_byte3, position_motor1_byte4, ...
%                        position_motor2_byte1, position_motor2_byte2, ...
%                        position_motor2_byte3, position_motor2_byte4];

%%%%%%%%%%%%%%%%%%%%%%%%%%%%%%%%%%%%%%%%%%%%%%%%%%%%%%%%%%
% save the running times of the three motors in a vector %
%%%%%%%%%%%%%%%%%%%%%%%%%%%%%%%%%%%%%%%%%%%%%%%%%%%%%%%%%%
% time_bytes_out = [time_motor0_byte1, time_motor0_byte2, ...
%                   time_motor0_byte3, time_motor1_byte1, ...
%                   time_motor1_byte2, time_motor1_byte3, ...
%                   time_motor2_byte1, time_motor2_byte2, time_motor2_byte3];

%%%%%%%%%%%%%%%%%%%%%%%%%%%%%%%%%%%%%%
% save values of digital input 0 - 3 %
%%%%%%%%%%%%%%%%%%%%%%%%%%%%%%%%%%%%%%
di03_bump_out = error_free_resp_out(32);

== matlab function KitGewerk2_v1_4/Robotino/receive direction, unit & velocity converter ==
  settings: sampleTime=dtpc/2
  data: direction_motor0_in input; v_x_out output; velocity_motor0_in input; direction_motor1_in input; velocity_motor1_in input; direction_motor2_in input; velocity_motor2_in input; v_y_out output; v_theta_out output
%%%%%%%%%%%%%%%%%%%%%%%%%%%%%%%%%%%%%%%%%%%%%%%%%%%%%%%%%%%%%%%%%%%%%%%%%%%
% assembly of the three separate positive motor velocities (resolution:   %
% 1Byte) and their rotation direction to positive and/or negative         %
% longitudinal, lateral & rotational velocities (in milimeters per        %
% second)                                                                 %
%                                                                         %
% inputs:  direction_motor0_in (rotating direction of motor0              %
%          (129 := counter-clockwise; 128 := clockwise)),                 %
%          velocity_motor0_in (from 0 to 255),                            %
%          direction_motor1_in (rotating direction of motor1              %
%          (0 := counter-clockwise; 1 := clockwise)),                     %
%          velocity_motor1_in (from 0 to 255),                            %
%          direction_motor2_in (rotating direction of motor2              %
%          (0 := counter-clockwise; 1 := clockwise)),                     %
%          velocity_motor2_in (from 0 to 255)                             %
% outputs: v_x_out (longitudinal velocity (in milimeters per second)),    %
%          v_y_out (lateral velocity (in milimeters per second)),         %
%          v_theta_out (rotational velocity (in milimeters per second))   %
%%%%%%%%%%%%%%%%%%%%%%%%%%%%%%%%%%%%%%%%%%%%%%%%%%%%%%%%%%%%%%%%%%%%%%%%%%%
function [v_x_out, v_y_out, v_theta_out] ...
    = fcn(direction_motor0_in, velocity_motor0_in, direction_motor1_in, ...
          velocity_motor1_in, direction_motor2_in, velocity_motor2_in)
%%%%%%%%%%%%%%%%%%%%%%%%%%%%%%%%%%%%%%%%%%%%%%%%%%%%%%%%%%%%%%%%%
% assembly of absolute motor velocity and rotating direction to %
% longitudinal, lateral & rotational velocity for every motor   %
%%%%%%%%%%%%%%%%%%%%%%%%%%%%%%%%%%%%%%%%%%%%%%%%%%%%%%%%%%%%%%%%%
if direction_motor0_in < 129
    v0 = -velocity_motor0_in;
else
    v0 =  velocity_motor0_in;
end

if direction_motor1_in < 1
    v1 = -velocity_motor1_in;
else
    v1 =  velocity_motor1_in;
end

if direction_motor2_in < 1
    v2 = -velocity_motor2_in;
else
    v2 =  velocity_motor2_in;
end

%%%%%%%%%%%%%%%%%%%%%%%%%%%%%%%%%%%%%%%%%%%%%%%%%%%%%%%%%%%%%%%%%%%%%%%%%
% conversion of the separate motor velocities from a value between -255 %
% and 255 to millimeters                                                %
%%%%%%%%%%%%%%%%%%%%%%%%%%%%%%%%%%%%%%%%%%%%%%%%%%%%%%%%%%%%%%%%%%%%%%%%%
f_rcv = 7.02;
v0    = v0 * f_rcv;
v1    = v1 * f_rcv;
v2    = v2 * f_rcv;

%%%%%%%%%%%%%%%%%%%%%%%%%%%%%%%%%%%%%%%%%%%%%%%%%%%%%%%%%%%%%%%%%%%%
% conversion from three separate motor velocities to longitudinal, %
% lateral & rotational velocity                                    %
%%%%%%%%%%%%%%%%%%%%%%%%%%%%%%%%%%%%%%%%%%%%%%%%%%%%%%%%%%%%%%%%%%%%
v_x_out     = (v2 - v0) / (2 * cosd(30));                         % in mm/s
v_y_out     = (v0 - 2 * v1 + v2) / 3;                             % in mm/s
v_theta_out = (v0 + v1 + v2) / (3 * 135);                        % in rad/s

== matlab function KitGewerk2_v1_4/Begrenzung ==
  data: win input; wout output
function wout = fnc(win)
wert= zeros(1);
if win > 500
    wert = 500;
else
    wert = win;
end
wout = wert;

== matlab function KitGewerk2_v1_4/Robotino/serial communication/stop by bumper ==
  settings: sampleTime=2*dtpc
  data: stop_out output; bumper input; stop_flag_in input; stop_flag_out output
%%%%%%%%%%%%%%%%%%%%%%%%%%%%%%%%%%%%%%%%%%%%%%%%%%%%%%%%%%%%%%%%%%%%%%%%%%%
% Recognition of collisions and creating of variables indicating and      %
% marking a collision                                                     %
%                                                                         %
% inputs: bumper (vector of the three bumper bytes)                       %
%         stop_flag_in (As long as no collision has occured,              %
%                       'stop_flag_in' contains the last bumper vector    %
%                       indicating no collision.                          %
%                       If a collision has occured, 'stop_flag_in'        %
%                       contains the last bumper vector indicating a      %
%                       collision until the simulation stops.)            %
% outputs: stop_out (indicates a collision: 1 = no collision;             %
%                                           0 = collision)                %
%          stop_flag_out (gets the actual bumper vector unless 'bumper'   %
%                         indicates no collision and 'stop_flag_in'       %
%                         indicates a past collision.)                    %
%%%%%%%%%%%%%%%%%%%%%%%%%%%%%%%%%%%%%%%%%%%%%%%%%%%%%%%%%%%%%%%%%%%%%%%%%%%
function [stop_out, stop_flag_out] = fcn(bumper, stop_flag_in)
if max(bumper) == 31       % as soon as the maximum value of the bumper ...
                              % vector indicates 31 a collision is detected
    stop_out = 0;
    stop_flag_out = bumper;
elseif max(stop_flag_in) == 31 % if the maximum value of 'stop_flag_in' ...
                                      % indicates a past collision (31) ...
    stop_out = 0;         % 'stop_out' gets 0 for a further stop of the ...
                                                           % motors and ...
    stop_flag_out = stop_flag_in; % 'stop_flag_out' gets the last bumper...
                                       % vector indicating a past collision
else                                                        % otherwise ...
    stop_out = 1;    % 'stop_out' gets 1 to keep the motors running and ...
    stop_flag_out = bumper; % 'stop_flag_out' gets the actual bumper vector
end

== matlab function KitGewerk2_v1_4/Robotino/distance converter ==
  settings: sampleTime=dtpc/2
  data: dms_in input; dms_out output
%%%%%%%%%%%%%%%%%%%%%%%%%%%%%%%%%%%%%%%%%%%%%%%%%%%%%%%%%%%%%%%%%%%%%%%%%%%
% conversion of the nine distance measuring sensor values (resolution:    %
% 1Byte) to unit milimeters (range: from 40mm to 1500mm) with linear      %
% interpolation                                                           %
%                                                                         %
% input:  vector containing the values of the nine distance measuring     %
%         sensors                                                         %
% output: vector containing the nine values in milimeters                 %
%%%%%%%%%%%%%%%%%%%%%%%%%%%%%%%%%%%%%%%%%%%%%%%%%%%%%%%%%%%%%%%%%%%%%%%%%%%
function dms_out = fcn(dms_in)

y_mm = [40, 45, 50, 60, 75, 100, 125, 150, 175, 200, 250, 300]; % , ...
        %400, 500, 600, 700, 800, 900, 1000, 1100, 1200, 1300, 1500];
    
x_sensor = [255, 249.7733813, 228.6082474, 193.6871795, ...
            152.0044843, 113.7266187, 92.42268041, ...
            76.36407767, 65.19289827, 55.1025641, ...
            43.06299213, 34.97068404]; % , 24.37410072, ...
            % 16.3381295, 11.62589928, 8.661870504, ...
            % 6.316546763, 4.74, 3.65, 2.96, 2.40, ...
            % 2.035971223, 1.539568345];

% x_sensor = round(100 * x_sensor) / 100;

dms_out = interp1(x_sensor, y_mm, dms_in, 'linear');
